simulink model "blocks"  (R2019a)
settings: Solver=VariableStepAuto  StartTime=0.0  StopTime=10.0  RelTol=1e-3
settings Model: Creator=adeye  LastModifiedBy=adeye

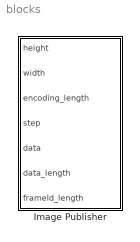
== system blocks ==
  Image Publisher : Subsystem  mask{topic='/camera_1/image_raw', message_type='sensor_msgs/Image', port=9090, timeout=2, frame_id='camera_1'}
      mask prompts: topic "Topic name"; message_type "Message type"; timeout "Timeout (s)"; frame_id "Frame id (keep '/default' if it's not used)"

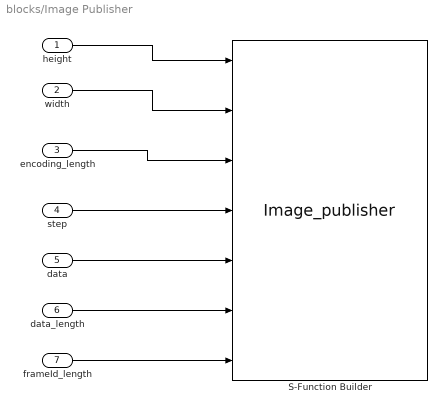
== system blocks/Image Publisher ==
  height : Inport
  width : Inport  Port=2
  encoding_length : Inport  Port=3
  step : Inport  Port=4
  data : Inport  Port=5
  data_length : Inport  Port=6
  frameId_length : Inport  Port=7
  S-Function Builder : S-Function  InitFcn=try, set_param(gcb,'FunctionName','Image_publisher'), end  FunctionName=Image_publisher  Parameters=int8(topic),int8(message_type),int8(frame_id),port,timeout  SFunctionModules=Image_publisher_wrapper rosbridge_functions  SFunctionDeploymentMode=off  EnableBusSupport=off  mask(S-Function Builder){}
      mask help: Simulink:masks:SFunctionBuilder_MD
      mask init:
      | val = [[.9  0.75 0.75 1 1 .9 .9 1]',[1 1 0.75 0.75 .9 .9 1 .9]'];try , sys = get_param(gcb,'SfunBuilderFcnName');if isempty(sys), sys = get_param(gcb,'FunctionName'); end,catch, sys = get_param(gcb,'FunctionName'); end
      settings: CopyFcn=set_param(gcbh,'LinkStatus','none')  PreSaveFcn=try, set_param(gcb,'FunctionName','Image_publisher'), end  OpenFcn=sfunctionwizard(gcbh)
      mask Display: plot(val(:,1),val(:,2)),disp(sys), port_label('input',1,'height'), port_label('input',2,'width'), port_label('input',3,'encoding_length'), port_label('input',4,'step'), port_label('input',5,'data'), port_label('input',6,'data_length'), port_label('input',7,'frameId_length')
  wires:
  height/1 -> S-Function Builder/1
  width/1 -> S-Function Builder/2
  encoding_length/1 -> S-Function Builder/3
  step/1 -> S-Function Builder/4
  data/1 -> S-Function Builder/5
  data_length/1 -> S-Function Builder/6
  frameId_length/1 -> S-Function Builder/7
